simulink model "Velo_Complet_BO"  (R2018a)
settings: Solver=VariableStepAuto  StartTime=0.0  StopTime=10.0  RelTol=1e-3
settings Model: Creator=chsira  LastModifiedBy=charl
settings DebuggingCC: LibraryContextMissingDiagnostic=warning
settings SFSimCC: SimUseLocalCustomCode=on
settings RTWCC: RTWUseLocalCustomCode=on

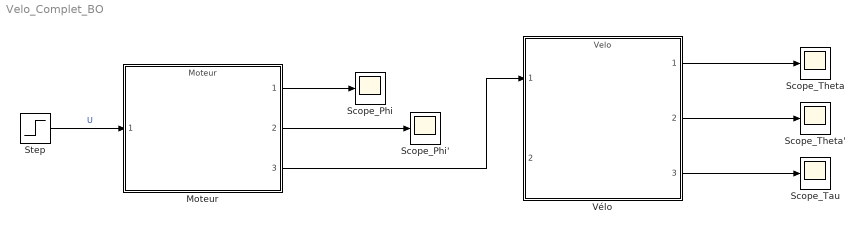
== system Velo_Complet_BO ==
  Moteur : ModelReference  ModelNameDialog=Moteur  SimulationMode=Normal  ModelReferenceVersion=1.16
  Scope_Phi : Scope
  Scope_Phi' : Scope
  Scope_Tau : Scope
  Scope_Theta : Scope
  Scope_Theta' : Scope
  Step : Step  Time=0  SampleTime=0
  Vélo : ModelReference  ModelNameDialog=Velo  ParameterArgumentNames=InitialCondition  ParameterArgumentValues=InitialCondition  UsingDefaultArgumentValue=0  SimulationMode=Normal  ModelReferenceVersion=1.22  InitialCondition=0  SimulationMode=Normal
  wires:
  Step/1 -> Moteur/1  "U"
  Moteur/1 -> Scope_Phi/1
  Moteur/2 -> Scope_Phi'/1
  Vélo/1 -> Scope_Theta/1
  Vélo/2 -> Scope_Theta'/1
  Moteur/3 -> Vélo/1
  Vélo/3 -> Scope_Tau/1
